simulink model "q22"  (R2019a)
settings: Solver=FixedStepAuto  StartTime=0.0  StopTime=0.1  FixedStep=1e-7  RelTol=1e-3
libraries: dsparch4 x2, simulink x1
settings Model: Creator=marco  LastModifiedBy=marco

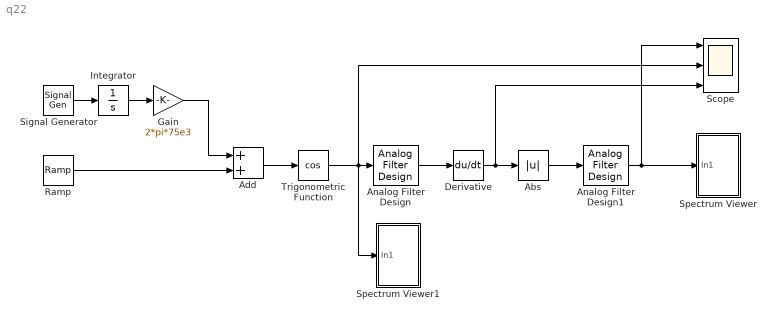
== system q22 ==
  Abs : Abs
  Add : Sum
  Analog Filter Design : dsparch4/Analog Filter Design  method=Butterworth  filttype=Bandpass  N=8  Wlo=2*pi*(1e6 - 1e4)  Whi=2*pi*(1e6 + 1e4)  Rp=2  Rs=40
  Analog Filter Design1 : dsparch4/Analog Filter Design  method=Butterworth  filttype=Lowpass  N=8  Wlo=2*pi*500e3  Whi=80  Rp=2  Rs=40
  Derivative : Derivative
  Gain : Gain  Gain=2*pi*75e3
  Integrator : Integrator
  Ramp : simulink/Sources/Ramp  slope=2*pi*(1e6)  start=0  InitialOutput=0
  Scope : Scope  NumInputPorts=3
  Signal Generator : SignalGenerator  WaveForm=square  Frequency=10e3
  Spectrum Viewer : Subsystem
  Spectrum Viewer1 : Subsystem
  Trigonometric Function : Trigonometry  Operator=cos
  wires:
  Add/1 -> Trigonometric Function/1
  Ramp/1 -> Add/2
  Signal Generator/1 -> Integrator/1
  Integrator/1 -> Gain/1
  Gain/1 -> Add/1
  Trigonometric Function/1 -> Scope/2, Spectrum Viewer1/1(In1), Analog Filter Design/1
  Analog Filter Design/1 -> Derivative/1
  Derivative/1 -> Scope/3, Abs/1
  Abs/1 -> Analog Filter Design1/1
  Analog Filter Design1/1 -> Scope/1, Spectrum Viewer/1(In1)

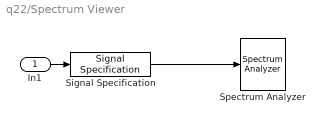
== system q22/Spectrum Viewer ==
  In1 : Inport
  Signal Specification : SignalSpecification  SampleTime=1e-7
  Spectrum Analyzer : SpectrumAnalyzer
  wires:
  In1/1 -> Signal Specification/1
  Signal Specification/1 -> Spectrum Analyzer/1

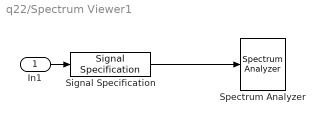
== system q22/Spectrum Viewer1 ==
  In1 : Inport
  Signal Specification : SignalSpecification  SampleTime=1e-7
  Spectrum Analyzer : SpectrumAnalyzer
  wires:
  In1/1 -> Signal Specification/1
  Signal Specification/1 -> Spectrum Analyzer/1
